simulink model "rtwdemo_fileprocess"  (Simulink 6.0)
settings: Solver=FixedStepDiscrete  StartTime=0.0  StopTime=48  FixedStep=1  RelTol=1e-3
libraries: rtwdemowidgets x2
settings Model: CovMetricSettings=d  Creator=The MathWorks Inc.  LastModifiedBy=batserve  ParamWorkspaceSource=ReferencedWorkspace  ExtModeTrigMode=oneshot  ExtModeArmWhenConnect=off  ExtModeAutoUpdateStatusClock=off
settings DataIOCC: LimitDataPoints=off  SaveFormat=StructureWithTime  SaveOutput=off  SaveTime=off  SignalLoggingName=sigsOut
settings OptimizationCC: InlineParams=on  EnforceIntegerDowncast=off  StateBitsets=on  DataBitsets=on  UseTempVars=on  ZeroExternalMemoryAtStartup=off  ZeroInternalMemoryAtStartup=off  InitFltsAndDblsToZero=off  NoFixptDivByZeroProtection=on  OptimizeModelRefInitCode=on  LifeSpan=1
settings DebuggingCC: CheckExecutionContextPreStartOutputMsg=on  CheckExecutionContextRuntimeOutputMsg=on  SolverPrmCheckMsg=none  IntegerOverflowMsg=none
settings ModelReferenceCC: UpdateModelReferenceTargets=IfOutOfDate
settings RTWCC: SystemTargetFile=ert.tlc  TLCOptions=-p0 -aWarnNonSaturatedBlocks=0  GenCodeOnly=on  TemplateMakefile=ert_default_tmf  GenerateReport=on  RTWVerbose=off  ProcessScript=ert_make_rtw_hook  IncludeHyperlinkInReport=on  LaunchReport=on
settings CodeAppCC: ForceParamTrailComments=on  IgnoreCustomStorageClasses=off  SimulinkDataObjDesc=on  PrefixModelToSubsysFcnNames=off  CustomSymbolStr=$N$M  InsertBlockDesc=on
settings ERTTargetCC: TargetFcnLib=ansi_tfl_tmw.mat  GenFloatMathFcnCalls=ANSI_C  IncludeMdlTerminateFcn=off  MultiInstanceERTCode=on  SupportNonFinite=off  SupportComplex=off  InlinedParameterPlacement=NonHierarchical  RootIOFormat=Individual Arguments  ERTCustomFileTemplate=rtwdemofileprocess.tlc  InitialValueSource=Model

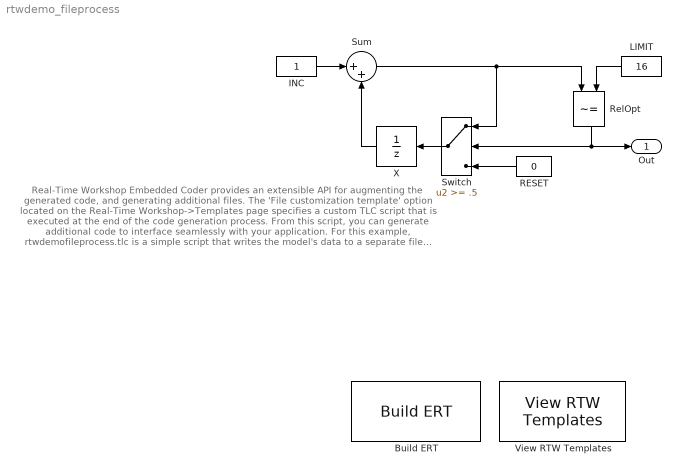
== system rtwdemo_fileprocess ==
  note: Real-Time Workshop Embedded Coder provides an extensible API for augmenting the generated
      | code, and generating additional files.  The 'File customization template' option located
      | on the Real-Time Workshop->Templates page specifies a custom TLC script that is executed
      | at the end of the code generation process.  From this script, you can generate additional
      | code to interface seamlessly with your application.
      |
      | For this example, rtwdemofileprocess.tlc is a simple script that writes the model's data
      | to a separate file model_data.c.  Do view the file, double-click the yellow button below
      | and press the Edit button to the right of the 'File customization template' option.
  Build ERT : rtwdemowidgets/Build ERT  attrib_overrides={'GenerateSampleERTMain','GenCodeOnly','ERTCustomFileTemplate','MultiInstanceERTCode'}
  INC : Constant  OutDataTypeMode=uint8
  LIMIT : Constant  Orientation=left  Value=16  OutDataTypeMode=uint8
  RESET : Constant  Orientation=left  Value=0  OutDataTypeMode=uint8
  RelOpt : RelationalOperator  Orientation=down  Operator=~=  InputSameDT=on
  Sum : Sum  Inputs=|++  InputSameDT=on
  Switch : Switch  Orientation=left  Threshold=.5  SaturateOnIntegerOverflow=on  InputSameDT=on
  View RTW Templates : rtwdemowidgets/View RTW Templates
  X : UnitDelay  Orientation=left  StateIdentifier=X
  Out : Outport
  wires:
  INC/1 -> Sum/1
  X/1 -> Sum/2
  Switch/1 -> X/1
  Sum/1 -> Switch/1, RelOpt/1
  LIMIT/1 -> RelOpt/2
  RESET/1 -> Switch/3
  RelOpt/1 -> Switch/2, Out/1
